simulink model "Simulink_Platoon"  (R2018b)
settings: Solver=VariableStepAuto  StartTime=0.0  StopTime=inf  RelTol=1e-3
values from neighbouring files (symbols this model uses):
  EgoName = block.DialogPrm(2).Data    [LeaderBlock.m]    (also in ObjectBlock.m; data_ver2.mat = ; data_ver2_2.mat = ; data_ver3.mat = )
  kT = block.DialogPrm(11).Data    [LeaderBlock.m]    (also in data_ver2.mat = [0.645779176886 6.55702927276]; data_ver3.mat = [0.22920630305 2.38997187052]; just_running.m = lqrd(A,b,Q,R,SumoTs))
  NumTLights = 0    [data_ver2.mat]    (also in data_ver3.mat; just_running.m)
  NumVehicles = block.DialogPrm(3).Data    [LeaderBlock.m]    (also in ObjectBlock.m; Untitled.m = 7; data_ver2.mat = 10; data_ver3.mat = 10)
  SensorRange = 200    [data_ver2.mat]    (also in data_ver3.mat; just_running.m)
  SumoCfg = 'data1\line.sumocfg'    [data_ver2.mat]    (also in data_ver3.mat; just_running.m)
  SumoGui = block.DialogPrm(7).Data    [LeaderBlock.m]    (also in data_ver2.mat = 1; data_ver3.mat = 1; just_running.m = 1)
  SumoIP = '127.0.0.1'    [data_ver2.mat]    (also in data_ver3.mat; just_running.m)
  SumoOptions = ''    [data_ver2.mat]    (also in data_ver3.mat; just_running.m)
  SumoPort = 8873    [data_ver2.mat]    (also in data_ver3.mat; just_running.m)
  SumoTs = block.DialogPrm(1).Data    [LeaderBlock.m]    (also in ObjectBlock.m; data_ver2.mat = 0.1; data_ver3.mat = 0.5; just_running.m = 0.5)
  V = block.DialogPrm(12).Data    [LeaderBlock.m]    (also in data_ver2.mat = 0.645779176886; data_ver3.mat = 0.22920630305; just_running.m = -1./(cT*inv(A-b*kT)*b); tet_ver1.m = zeros(length(x),length(y)))
settings Model: Creator=HP  LastModifiedBy=HP

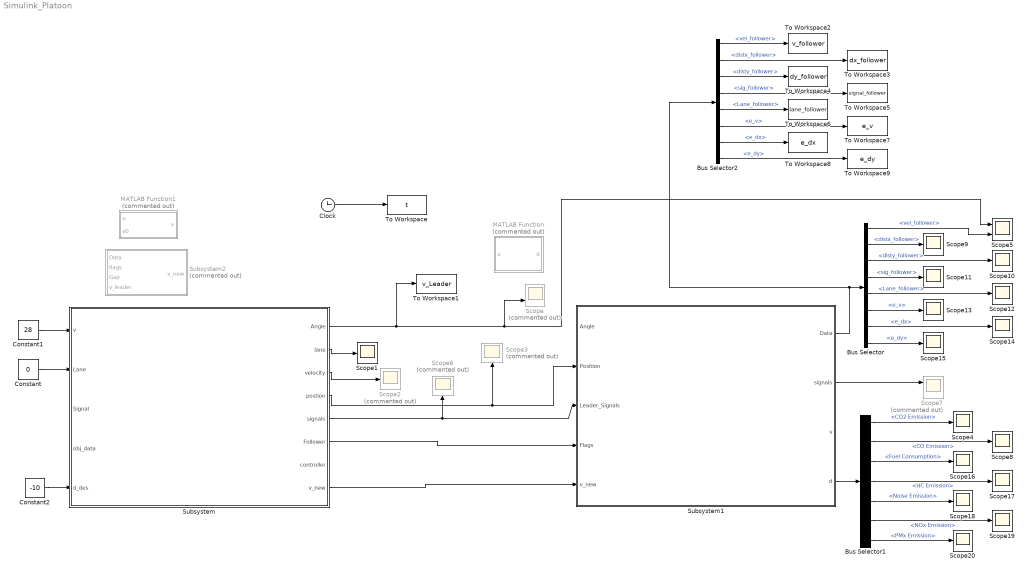
== system Simulink_Platoon ==
  Bus Selector : BusSelector  OutputSignals=vel_follower,distx_follower,disty_follower,sig_follower,Lane_follower,e_v,e_dx,e_dy
  Bus Selector1 : BusSelector  OutputSignals=CO2 Emission,CO Emission,Fuel Consumption,HC Emission,Noise Emission,NOx Emission,PMx Emission
  Bus Selector2 : BusSelector  OutputSignals=vel_follower,distx_follower,disty_follower,sig_follower,Lane_follower,e_v,e_dx,e_dy
  Clock : Clock
  Constant : Constant  Value=0
  Constant1 : Constant  Value=28
  Constant2 : Constant  Value=-10
  MATLAB Function : MATLAB Function  Commented=on  TreatAsAtomicUnit=on
  MATLAB Function1 : MATLAB Function  Commented=on  TreatAsAtomicUnit=on
  Scope : Scope  Commented=on  NumInputPorts=2
  Scope{1,4,8..20} (15 alike) : Scope
  Scope2 : Scope  Commented=on
  Scope3 : Scope  Commented=on
  Scope5 : Scope  NumInputPorts=2
  Scope6 : Scope  Commented=on
  Scope7 : Scope  Commented=on  NumInputPorts=2
  Subsystem : Subsystem
  Subsystem1 : Subsystem
  Subsystem2 : Subsystem  Commented=on
  To Workspace : ToWorkspace  VariableName=t  SampleTime=SumoTs
  To Workspace1 : ToWorkspace  VariableName=v_Leader  SampleTime=-1
  To Workspace2 : ToWorkspace  VariableName=v_follower  SampleTime=SumoTs
  To Workspace3 : ToWorkspace  VariableName=dx_follower  SampleTime=SumoTs
  To Workspace4 : ToWorkspace  VariableName=dy_follower  SampleTime=SumoTs
  To Workspace5 : ToWorkspace  VariableName=signal_follower  SampleTime=SumoTs
  To Workspace6 : ToWorkspace  VariableName=lane_follower  SampleTime=SumoTs
  To Workspace7 : ToWorkspace  VariableName=e_v  SampleTime=SumoTs
  To Workspace8 : ToWorkspace  VariableName=e_dx  SampleTime=SumoTs
  To Workspace9 : ToWorkspace  VariableName=e_dy  SampleTime=SumoTs
  wires:
  Subsystem/1(Angle) -> To Workspace1/1, Scope5/1, Scope/2
  Subsystem/2(lane) -> Scope1/1
  Subsystem/3(velocity) -> Scope2/1
  Constant/1 -> Subsystem/2(Lane)
  Constant1/1 -> Subsystem/1(v)
  Subsystem1/1(Data) -> Bus Selector/1, Bus Selector2/1
  Subsystem/6(Follower) -> Subsystem1/4(Flags)
  Subsystem/4(postion) -> Scope3/1, Subsystem1/2(Position)
  Subsystem/5(signals) -> Subsystem1/3(Leader_Signals), Scope6/1
  Subsystem1/2(signals) -> Scope7/1
  Subsystem/8(v_new) -> Subsystem1/5(v_new)
  Bus Selector/4 -> Scope11/1  "<sig_follower>"
  Bus Selector/1 -> Scope5/2  "<vel_follower>"
  Bus Selector/2 -> Scope9/1  "<distx_follower>"
  Bus Selector/3 -> Scope10/1  "<disty_follower>"
  Bus Selector/5 -> Scope12/1  "<Lane_follower>"
  Bus Selector/6 -> Scope13/1  "<e_v>"
  Bus Selector/7 -> Scope14/1  "<e_dx>"
  Bus Selector/8 -> Scope15/1  "<e_dy>"
  Constant2/1 -> Subsystem/5(d_des)
  Subsystem1/4(d) -> Bus Selector1/1
  Bus Selector1/1 -> Scope4/1  "<CO2 Emission>"
  Bus Selector1/2 -> Scope8/1  "<CO Emission>"
  Bus Selector1/3 -> Scope16/1  "<Fuel Consumption>"
  Bus Selector1/4 -> Scope17/1  "<HC Emission>"
  Bus Selector1/5 -> Scope18/1  "<Noise Emission>"
  Bus Selector1/6 -> Scope19/1  "<NOx Emission>"
  Bus Selector1/7 -> Scope20/1  "<PMx Emission>"
  Clock/1 -> To Workspace/1
  Bus Selector2/1 -> To Workspace2/1  "<vel_follower>"
  Bus Selector2/2 -> To Workspace3/1  "<distx_follower>"
  Bus Selector2/3 -> To Workspace4/1  "<disty_follower>"
  Bus Selector2/4 -> To Workspace5/1  "<sig_follower>"
  Bus Selector2/5 -> To Workspace6/1  "<Lane_follower>"
  Bus Selector2/6 -> To Workspace7/1  "<e_v>"
  Bus Selector2/7 -> To Workspace8/1  "<e_dx>"
  Bus Selector2/8 -> To Workspace9/1  "<e_dy>"

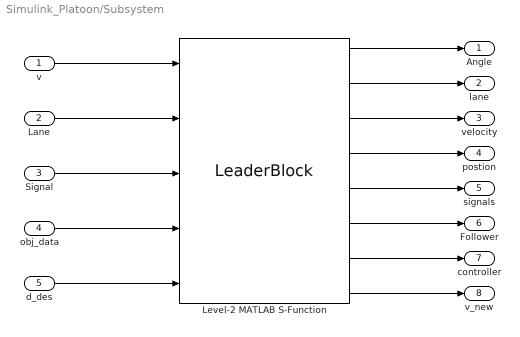
== system Simulink_Platoon/Subsystem ==
  v : Inport
  Lane : Inport  Port=2
  Signal : Inport  Port=3
  obj_data : Inport  Port=4
  d_des : Inport  Port=5
  Level-2 MATLAB S-Function : M-S-Function  FunctionName=LeaderBlock  Parameters=SumoTs,EgoName,NumVehicles,SumoCfg,SumoIP,SumoPort,SumoGui,SumoOptions,NumTLights,SensorRange,kT,V
  Angle : Outport
  lane : Outport  Port=2
  velocity : Outport  Port=3
  postion : Outport  Port=4
  signals : Outport  Port=5
  Follower : Outport  Port=6
  controller : Outport  Port=7
  v_new : Outport  Port=8
  wires:
  Signal/1 -> Level-2 MATLAB S-Function/3
  v/1 -> Level-2 MATLAB S-Function/1
  Lane/1 -> Level-2 MATLAB S-Function/2
  Level-2 MATLAB S-Function/1 -> Angle/1
  Level-2 MATLAB S-Function/2 -> lane/1
  Level-2 MATLAB S-Function/3 -> velocity/1
  Level-2 MATLAB S-Function/4 -> postion/1
  Level-2 MATLAB S-Function/5 -> signals/1
  obj_data/1 -> Level-2 MATLAB S-Function/4
  Level-2 MATLAB S-Function/6 -> Follower/1
  Level-2 MATLAB S-Function/7 -> controller/1
  Level-2 MATLAB S-Function/8 -> v_new/1
  d_des/1 -> Level-2 MATLAB S-Function/5

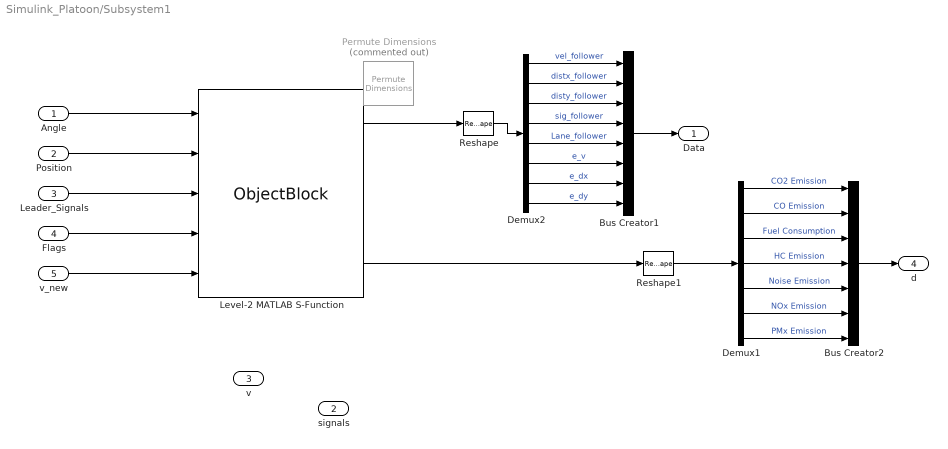
== system Simulink_Platoon/Subsystem1 ==
  Angle : Inport
  Position : Inport  Port=2
  Leader_Signals : Inport  Port=3
  Flags : Inport  Port=4
  v_new : Inport  Port=5
  Bus Creator1 : BusCreator  Inputs=8
  Bus Creator2 : BusCreator  Inputs=7
  Demux1 : Demux  Outputs=[-1,-1,-1,-1,-1,-1,-1]
  Demux2 : Demux  Outputs=[-1,-1,-1,-1,-1,-1,-1,-1]
  Level-2 MATLAB S-Function : M-S-Function  FunctionName=ObjectBlock  Parameters=SumoTs,EgoName,NumVehicles,SumoCfg,SumoIP,SumoPort,SumoGui,SumoOptions,NumTLights,SensorRange
  Permute Dimensions : PermuteDimensions  Commented=on
  Reshape : Reshape
  Reshape1 : Reshape
  Data : Outport
  signals : Outport  Port=2
  v : Outport  Port=3
  d : Outport  Port=4
  wires:
  Angle/1 -> Level-2 MATLAB S-Function/1
  Position/1 -> Level-2 MATLAB S-Function/2
  Level-2 MATLAB S-Function/1 -> Reshape/1
  Reshape/1 -> Demux2/1
  Demux2/1 -> Bus Creator1/1  "vel_follower"
  Demux2/2 -> Bus Creator1/2  "distx_follower"
  Bus Creator1/1 -> Data/1
  Leader_Signals/1 -> Level-2 MATLAB S-Function/3
  Flags/1 -> Level-2 MATLAB S-Function/4
  v_new/1 -> Level-2 MATLAB S-Function/5
  Demux2/3 -> Bus Creator1/3  "disty_follower"
  Demux2/4 -> Bus Creator1/4  "sig_follower"
  Demux2/5 -> Bus Creator1/5  "Lane_follower"
  Demux2/6 -> Bus Creator1/6  "e_v"
  Demux2/7 -> Bus Creator1/7  "e_dx"
  Demux2/8 -> Bus Creator1/8  "e_dy"
  Demux1/1 -> Bus Creator2/1  "CO2 Emission"
  Bus Creator2/1 -> d/1
  Demux1/7 -> Bus Creator2/7  "PMx Emission"
  Demux1/2 -> Bus Creator2/2  "CO Emission"
  Demux1/6 -> Bus Creator2/6  "NOx Emission"
  Demux1/4 -> Bus Creator2/4  "HC Emission"
  Demux1/3 -> Bus Creator2/3  "Fuel Consumption"
  Demux1/5 -> Bus Creator2/5  "Noise Emission"
  Reshape1/1 -> Demux1/1
  Level-2 MATLAB S-Function/3 -> Reshape1/1

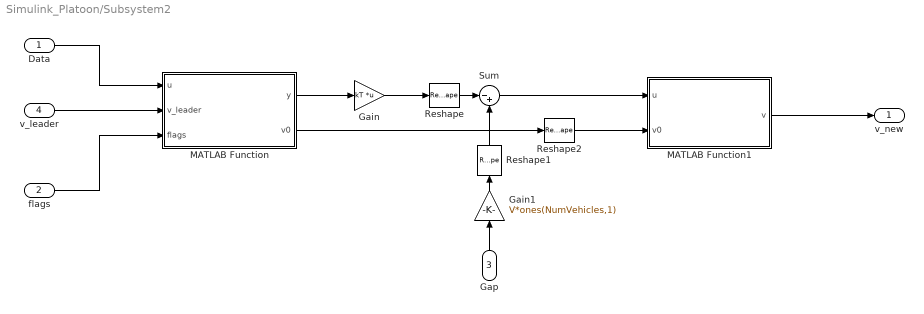
== system Simulink_Platoon/Subsystem2 ==
  Data : Inport
  flags : Inport  Port=2
  Gap : Inport  Port=3
  v_leader : Inport  Port=4
  Gain : Gain  Gain=kT  Multiplication=Matrix(K*u)
  Gain1 : Gain  Gain=V*ones(NumVehicles,1)
  MATLAB Function : MATLAB Function  TreatAsAtomicUnit=on
  MATLAB Function1 : MATLAB Function  TreatAsAtomicUnit=on
  Reshape : Reshape
  Reshape1 : Reshape
  Reshape2 : Reshape
  Sum : Sum  Inputs=|-+
  v_new : Outport
  wires:
  Data/1 -> MATLAB Function/1(u)
  flags/1 -> MATLAB Function/3(flags)
  MATLAB Function/1(y) -> Gain/1
  Gain/1 -> Reshape/1
  Gain1/1 -> Reshape1/1
  Gap/1 -> Gain1/1
  Sum/1 -> MATLAB Function1/1(u)
  MATLAB Function/2(v0) -> Reshape2/1
  MATLAB Function1/1(v) -> v_new/1
  v_leader/1 -> MATLAB Function/2(v_leader)
  Reshape/1 -> Sum/1
  Reshape1/1 -> Sum/2
  Reshape2/1 -> MATLAB Function1/2(v0)

== matlab function Simulink_Platoon/Subsystem2/MATLAB Function1 ==
  data: u input; v output; v0 input; SumoTs parameter
function v = fcn(u,v0,SumoTs)

v = u*SumoTs + v0;

== matlab function Simulink_Platoon/Subsystem2/MATLAB Function ==
  data: u input; v_leader input; y output; flags input; v0 output
function [y,v0] = fcn(u,v_leader,flags)

v  = u(1,:);
dx = u(2,:);
dy = u(3,:);

edx = zeros(length(v),1);
edy = zeros(length(v),1);
ev  = zeros(length(v),1);
ed  = zeros(length(v),1);

% v0 = zeros(1,NumVehicles);
% y  = zeros(2,NumVehicles);

idx = find(flags);
if ~isempty(idx)
    d = sqrt(dx(idx).^2 + dy(idx).^2);
    [dist,sortIdx] = sort(d);
    temp = idx(sortIdx);
    switch length(temp)
        case 1
            edx(temp) = dx(temp);
            edy(temp) = dy(temp);
            ev(temp)  = v(temp) - v_leader;
            ed  = -sqrt(edx.^2 + edy.^2);
        otherwise
            edx(temp(1)) = dx(temp(1));
            edy(temp(1)) = dy(temp(1));
            edx([temp(2:end)]) = dx([temp(2:end)]) - dx([temp(1:end-1)]);
            edy([temp(2:end)]) = dy([temp(2:end)]) - dy([temp(1:end-1)]);
            
            ev(temp(1)) = v(temp(1)) - v_leader;
            ev([temp(2:end)]) = v([temp(2:end)]) - v([temp(1:end-1)]);

            ed  = -sqrt(edx.^2 + edy.^2);
    end
end
y = [ed,ev]';
v0 = v;

== matlab function Simulink_Platoon/MATLAB Function1 ==
  data: u input; v output; v0 input; SumoTs parameter
function v = fcn(u,v0,SumoTs)

v = u*SumoTs + v0;

== matlab function Simulink_Platoon/MATLAB Function ==
  data: u input; d output
function d  = fcn(u)

v  = u(1,:);
dx = u(2,:);
dy = u(3,:);

d = -sqrt(dx.^2+dy.^2);
